simulink model "GuytonModel1972_R2018"  (R2018a)
settings: Solver=ode23tb  StartTime=0.0  StopTime=2e6  MaxStep=90  RelTol=1e-3  EnableMultiTasking=on
(part 2 of 2)

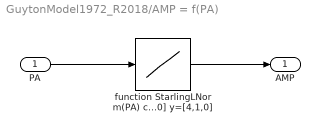
== system GuytonModel1972_R2018/AMP = f(PA) ==
  PA : Inport
  function StarlingLNorm(PA) cubic spline interpolation x=[0,100,200] y=[4,1,0] : Lookup_n-D  NumberOfTableDimensions=1  BreakpointsForDimension1=[0,100,200]  Table=[4,1,0]  ExtrapMethod=Clip  DiagnosticForOutOfRangeInput=Warning  UseLastTableValue=on  InputSameDT=on
  AMP : Outport
  wires:
  PA/1 -> function StarlingLNorm(PA) cubic spline interpolation x=[0,100,200] y=[4,1,0]/1
  function StarlingLNorm(PA) cubic spline interpolation x=[0,100,200] y=[4,1,0]/1 -> AMP/1

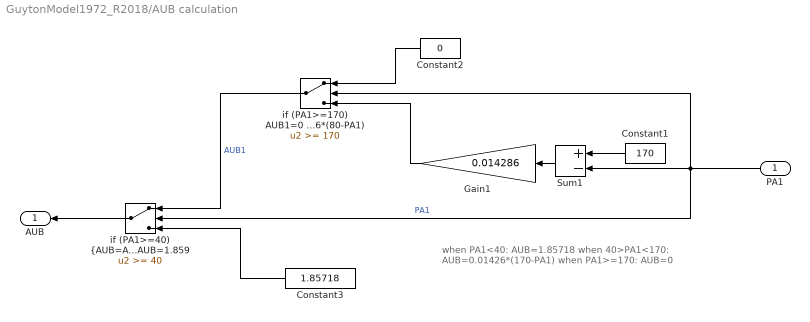
== system GuytonModel1972_R2018/AUB calculation ==
  note: when PA1<40:            AUB=1.85718
      | when  40>PA1<170:  AUB=0.01426*(170-PA1)
      | when PA1>=170:        AUB=0
  PA1 : Inport
  Constant1 : Constant  Value=170
  Constant2 : Constant  Value=0
  Constant3 : Constant  Value=1.85718
  Gain1 : Gain  Gain=0.014286  SaturateOnIntegerOverflow=on  OutDataTypeStr=Inherit: Same as input  ParamDataTypeStr=Inherit: Same as input
  Sum1 : Sum  Inputs=+-  SaturateOnIntegerOverflow=on  InputSameDT=on  OutDataTypeStr=Inherit: Same as first input
  if (PA1>=170) AUB1=0 else AUB1=0.014286*(80-PA1) : Switch  Threshold=170  SaturateOnIntegerOverflow=on  InputSameDT=on
  "if (PA1>=40) {AUB=AUB1) else AUB=1.859" : Switch  Threshold=40  SaturateOnIntegerOverflow=on  InputSameDT=on
  AUB : Outport  InitialOutput=0
  wires:
  "if (PA1>=40) {AUB=AUB1) else AUB=1.859"/1 -> AUB/1
  Constant3/1 -> "if (PA1>=40) {AUB=AUB1) else AUB=1.859"/3
  if (PA1>=170) AUB1=0 else AUB1=0.014286*(80-PA1)/1 -> "if (PA1>=40) {AUB=AUB1) else AUB=1.859"/1  "AUB1"
  Constant2/1 -> if (PA1>=170) AUB1=0 else AUB1=0.014286*(80-PA1)/1
  Gain1/1 -> if (PA1>=170) AUB1=0 else AUB1=0.014286*(80-PA1)/3
  PA1/1 -> "if (PA1>=40) {AUB=AUB1) else AUB=1.859"/2, if (PA1>=170) AUB1=0 else AUB1=0.014286*(80-PA1)/2, Sum1/2  "PA1"
  Sum1/1 -> Gain1/1
  Constant1/1 -> Sum1/1

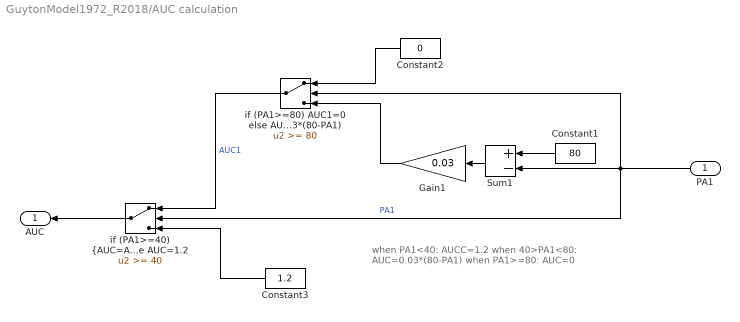
== system GuytonModel1972_R2018/AUC calculation ==
  note: when PA1<40:          AUCC=1.2
      | when  40>PA1<80:  AUC=0.03*(80-PA1)
      | when PA1>=80:        AUC=0
  PA1 : Inport
  Constant1 : Constant  Value=80
  Constant2 : Constant  Value=0
  Constant3 : Constant  Value=1.2
  Gain1 : Gain  Gain=0.03  SaturateOnIntegerOverflow=on  OutDataTypeStr=Inherit: Same as input  ParamDataTypeStr=Inherit: Same as input
  Sum1 : Sum  Inputs=+-  SaturateOnIntegerOverflow=on  InputSameDT=on  OutDataTypeStr=Inherit: Same as first input
  "if (PA1>=40) {AUC=AUC1) else AUC=1.2" : Switch  Threshold=40  SaturateOnIntegerOverflow=on  InputSameDT=on
  if (PA1>=80) AUC1=0 else AUC1=0.03*(80-PA1) : Switch  Threshold=80  SaturateOnIntegerOverflow=on  InputSameDT=on
  AUC : Outport  InitialOutput=0
  wires:
  Constant1/1 -> Sum1/1
  Sum1/1 -> Gain1/1
  PA1/1 -> Sum1/2, if (PA1>=80) AUC1=0 else AUC1=0.03*(80-PA1)/2, "if (PA1>=40) {AUC=AUC1) else AUC=1.2"/2  "PA1"
  Gain1/1 -> if (PA1>=80) AUC1=0 else AUC1=0.03*(80-PA1)/3
  Constant2/1 -> if (PA1>=80) AUC1=0 else AUC1=0.03*(80-PA1)/1
  if (PA1>=80) AUC1=0 else AUC1=0.03*(80-PA1)/1 -> "if (PA1>=40) {AUC=AUC1) else AUC=1.2"/1  "AUC1"
  Constant3/1 -> "if (PA1>=40) {AUC=AUC1) else AUC=1.2"/3
  "if (PA1>=40) {AUC=AUC1) else AUC=1.2"/1 -> AUC/1

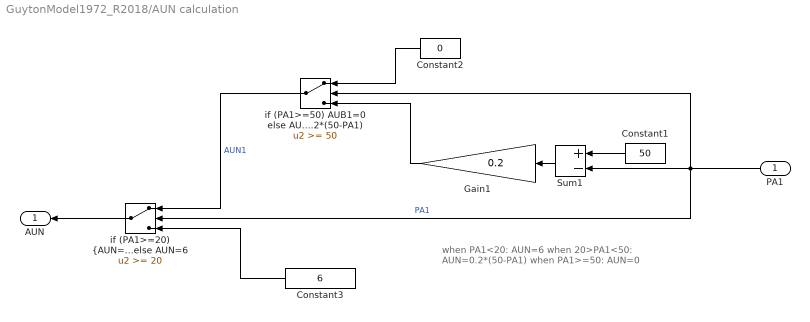
== system GuytonModel1972_R2018/AUN calculation ==
  note: when PA1<20:           AUN=6
      | when  20>PA1<50:  AUN=0.2*(50-PA1)
      | when PA1>=50:        AUN=0
  PA1 : Inport
  Constant1 : Constant  Value=50
  Constant2 : Constant  Value=0
  Constant3 : Constant  Value=6
  Gain1 : Gain  Gain=0.2  SaturateOnIntegerOverflow=on  OutDataTypeStr=Inherit: Same as input  ParamDataTypeStr=Inherit: Same as input
  Sum1 : Sum  Inputs=+-  SaturateOnIntegerOverflow=on  InputSameDT=on  OutDataTypeStr=Inherit: Same as first input
  "if (PA1>=20) {AUN=AUN1) else AUN=6" : Switch  Threshold=20  SaturateOnIntegerOverflow=on  InputSameDT=on
  if (PA1>=50) AUB1=0 else AUN1=0.2*(50-PA1) : Switch  Threshold=50  SaturateOnIntegerOverflow=on  InputSameDT=on
  AUN : Outport  InitialOutput=0
  wires:
  Constant1/1 -> Sum1/1
  Sum1/1 -> Gain1/1
  PA1/1 -> Sum1/2, if (PA1>=50) AUB1=0 else AUN1=0.2*(50-PA1)/2, "if (PA1>=20) {AUN=AUN1) else AUN=6"/2  "PA1"
  Gain1/1 -> if (PA1>=50) AUB1=0 else AUN1=0.2*(50-PA1)/3
  Constant2/1 -> if (PA1>=50) AUB1=0 else AUN1=0.2*(50-PA1)/1
  if (PA1>=50) AUB1=0 else AUN1=0.2*(50-PA1)/1 -> "if (PA1>=20) {AUN=AUN1) else AUN=6"/1  "AUN1"
  Constant3/1 -> "if (PA1>=20) {AUN=AUN1) else AUN=6"/3
  "if (PA1>=20) {AUN=AUN1) else AUN=6"/1 -> AUN/1

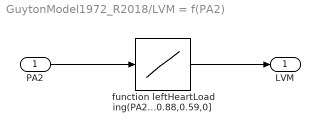
== system GuytonModel1972_R2018/LVM = f(PA2) ==
  PA2 : Inport
  "function leftHeartLoading(PA2) cubic spline interpolation x=[0,100, 125, 160, 200, 240] y=[1.04, 1.0,0.97,0.88,0.59,0]" : Lookup_n-D  NumberOfTableDimensions=1  BreakpointsForDimension1=[0,70, 100,125, 160, 200, 240]  Table=[1.04, 1.025, 1.0,0.97,0.88,0.59,0]  ExtrapMethod=Clip  UseLastTableValue=on  InputSameDT=on
  LVM : Outport
  wires:
  "function leftHeartLoading(PA2) cubic spline interpolation x=[0,100, 125, 160, 200, 240] y=[1.04, 1.0,0.97,0.88,0.59,0]"/1 -> LVM/1
  PA2/1 -> "function leftHeartLoading(PA2) cubic spline interpolation x=[0,100, 125, 160, 200, 240] y=[1.04, 1.0,0.97,0.88,0.59,0]"/1

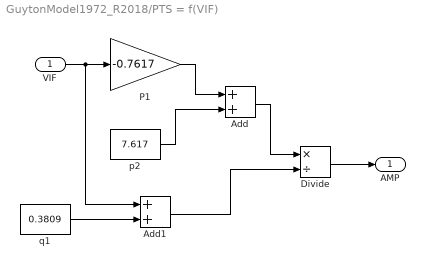
== system GuytonModel1972_R2018/PTS = f(VIF) ==
  VIF : Inport
  Add : Sum
  Add1 : Sum
  Divide : Product  Inputs=*/
  P1 : Gain  Gain=-0.7617
  p2 : Constant  Value=7.617
  q1 : Constant  Value=0.3809
  AMP : Outport
  wires:
  Divide/1 -> AMP/1
  Add/1 -> Divide/1
  Add1/1 -> Divide/2
  q1/1 -> Add1/2
  P1/1 -> Add/1
  p2/1 -> Add/2
  VIF/1 -> Add1/1, P1/1

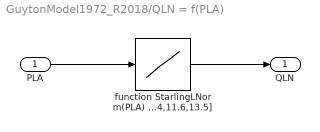
== system GuytonModel1972_R2018/QLN = f(PLA) ==
  PLA : Inport
  function StarlingLNorm(PLA) cubic spline interpolation x=[-4.5,-4,0,-1,3,6,10] y=[0,0.01,3.6,5.05,9.4,11.6,13.5] : Lookup_n-D  NumberOfTableDimensions=1  BreakpointsForDimension1=[-10,-9,-8,-7,-6,-5,-4.5,-4, -1,0, 3, 6, 10,11,12,13,15]  Table=[0,0,0,0,0,0,0,0.01, 3.6,5.05, 9.4, 11.6,13.5, 13.5, 13.5, 13.5,13.5]  ExtrapMethod=Clip  UseLastTableValue=on  InputSameDT=on
  QLN : Outport
  wires:
  PLA/1 -> function StarlingLNorm(PLA) cubic spline interpolation x=[-4.5,-4,0,-1,3,6,10] y=[0,0.01,3.6,5.05,9.4,11.6,13.5]/1
  function StarlingLNorm(PLA) cubic spline interpolation x=[-4.5,-4,0,-1,3,6,10] y=[0,0.01,3.6,5.05,9.4,11.6,13.5]/1 -> QLN/1

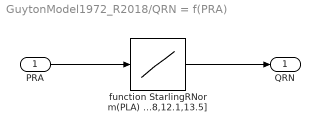
== system GuytonModel1972_R2018/QRN = f(PRA) ==
  PRA : Inport
  function StarlingRNorm(PLA) cubic spline interpolation x=[-6,-3,-1,0,2,4,8] y=[0,0.75,2.6,5.0,9.8,12.1,13.5] : Lookup_n-D  NumberOfTableDimensions=1  BreakpointsForDimension1=[-10,-9, -8,-7,-6, -3, -1, 2, 4, 8,8.5, 9,10,11,12,13]  Table=[0,0, 0,0,0,0.75,2.6,9.8,12.1,13.5,13.5,13.5,13.5,13.5,13.5,13.5]  ExtrapMethod=Clip  UseLastTableValue=on  InputSameDT=on
  QRN : Outport
  wires:
  function StarlingRNorm(PLA) cubic spline interpolation x=[-6,-3,-1,0,2,4,8] y=[0,0.75,2.6,5.0,9.8,12.1,13.5]/1 -> QRN/1
  PRA/1 -> function StarlingRNorm(PLA) cubic spline interpolation x=[-6,-3,-1,0,2,4,8] y=[0,0.75,2.6,5.0,9.8,12.1,13.5]/1

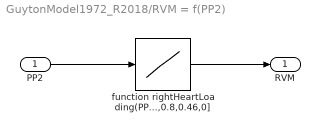
== system GuytonModel1972_R2018/RVM = f(PP2) ==
  PP2 : Inport
  function rightHeartLoading(PP2) cubic spline interpolation x=[-0,-20,24,30,38,45] y=[1.06,0.97,0.93,0.8,0.46,0] : Lookup_n-D  NumberOfTableDimensions=1  BreakpointsForDimension1=[0,10,20, 24, 30, 38, 45]  Table=[1.06,1.03, 0.97,0.93,0.8,0.46,0]  ExtrapMethod=Clip  UseLastTableValue=on  InputSameDT=on
  RVM : Outport
  wires:
  function rightHeartLoading(PP2) cubic spline interpolation x=[-0,-20,24,30,38,45] y=[1.06,0.97,0.93,0.8,0.46,0]/1 -> RVM/1
  PP2/1 -> function rightHeartLoading(PP2) cubic spline interpolation x=[-0,-20,24,30,38,45] y=[1.06,0.97,0.93,0.8,0.46,0]/1
